simulink model "hydro2pumps_iov1"  (Simulink 7.4)
settings: Solver=ode1  StartTime=0.0  StopTime=inf  FixedStep=0.5  RelTol=1e-3  AbsTol=1e-6
libraries: hydro2pumps_lib x1
settings Model: Creator=dmedonza  LastModifiedBy=student
settings DataIOCC: LimitDataPoints=off  SignalLoggingName=sigsOut
settings OptimizationCC: BooleanDataType=off
settings DebuggingCC: SaveWithParameterizedLinksMsg=none  SignalResolutionControl=TryResolveAllWithWarning  SolverPrmCheckMsg=none  MultiTaskDSMMsg=warning  MultiTaskCondExecSysMsg=none  StrictBusMsg=None
settings HardwareCC: TargetUnknown=on
settings RTWCC: TemplateMakefile=grt_vc.tmf  IncludeERTFirstTime=on

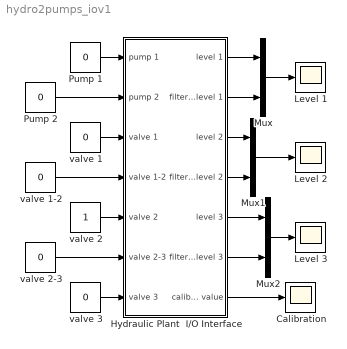
== system hydro2pumps_iov1 ==
  Calibration : Scope
      settings: TickLabels=on  TimeRange=20  YMin=0  YMax=100  SaveName=l3  DataFormat=Array
  Hydraulic Plant  I/O Interface : Subsystem
      mask Display: disp('Two Pumps\nHydraulic\nPlant\nI/O Interface')
  Level 1 : Scope
      settings: TickLabels=on  TimeRange=20  YMin=0  YMax=100  SaveName=l1  DataFormat=Array
  Level 2 : Scope
      settings: TickLabels=on  TimeRange=20  YMin=0  YMax=100  SaveName=l2  DataFormat=Array
  Level 3 : Scope
      settings: TickLabels=on  TimeRange=20  YMin=0  YMax=100  SaveName=lx  DataFormat=Array
  Mux : Mux  Inputs=2
  Mux1 : Mux  Inputs=2
  Mux2 : Mux  Inputs=2
  Pump 1 : Constant  Value=0  OutDataType=sfix(16)  OutScaling=2^0
  Pump 2 : Constant  Value=0  OutDataType=sfix(16)  OutScaling=2^0
  "valve 1 " : Constant  Value=0  OutDataType=sfix(16)  OutScaling=2^0
  valve 1-2 : Constant  Value=0  OutDataType=sfix(16)  OutScaling=2^0
  valve 2 : Constant  OutDataType=sfix(16)  OutScaling=2^0
  valve 2-3 : Constant  Value=0  OutDataType=sfix(16)  OutScaling=2^0
  valve 3 : Constant  Value=0  OutDataType=sfix(16)  OutScaling=2^0
  wires:
  Mux/1 -> Level 1/1
  Mux2/1 -> Level 3/1
  Pump 1/1 -> Hydraulic Plant  I/O Interface/1(pump 1)
  Pump 2/1 -> Hydraulic Plant  I/O Interface/2(pump 2)
  "valve 1 "/1 -> Hydraulic Plant  I/O Interface/3(valve 1)
  valve 1-2/1 -> Hydraulic Plant  I/O Interface/4(valve 1-2)
  valve 2/1 -> Hydraulic Plant  I/O Interface/5(valve 2)
  valve 2-3/1 -> Hydraulic Plant  I/O Interface/6(valve 2-3)
  valve 3/1 -> Hydraulic Plant  I/O Interface/7(valve 3)
  Hydraulic Plant  I/O Interface/1(level 1) -> Mux/1
  Hydraulic Plant  I/O Interface/2(filtered level 1) -> Mux/2
  Hydraulic Plant  I/O Interface/3(level 2) -> Mux1/1
  Hydraulic Plant  I/O Interface/4(filtered level 2) -> Mux1/2
  Hydraulic Plant  I/O Interface/5(level 3) -> Mux2/1
  Hydraulic Plant  I/O Interface/6(filtered level 3) -> Mux2/2
  Hydraulic Plant  I/O Interface/7(calibration value) -> Calibration/1
  Mux1/1 -> Level 2/1

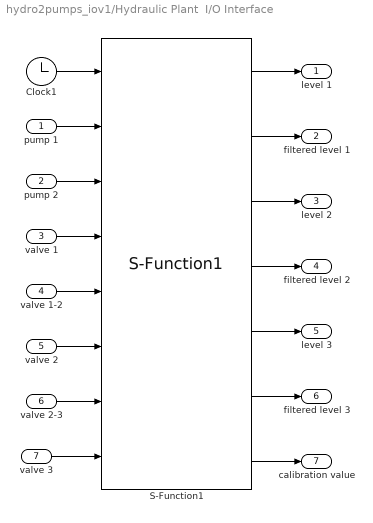
== system hydro2pumps_iov1/Hydraulic Plant  I/O Interface ==
  pump 1 : Inport  OutDataType=sfix(16)  OutScaling=2^0
  pump 2 : Inport  Port=2  OutDataType=sfix(16)  OutScaling=2^0
  valve 1 : Inport  Port=3  OutDataType=sfix(16)  OutScaling=2^0
  valve 1-2 : Inport  Port=4  OutDataType=sfix(16)  OutScaling=2^0
  valve 2 : Inport  Port=5  OutDataType=sfix(16)  OutScaling=2^0
  valve 2-3 : Inport  Port=6  OutDataType=sfix(16)  OutScaling=2^0
  valve 3 : Inport  Port=7  OutDataType=sfix(16)  OutScaling=2^0
  Clock1 : Clock
      settings: Decimation=10
  S-Function1 : hydro2pumps_lib/S-Function1  Priority=1  com_port=COM4  Ts=0.5  events_ot=2  rd_timeout=250  matlab_prior=ABOVE_NORMAL_PRIORITY  warning=on  printout=off
  level 1 : Outport
  filtered level 1 : Outport  Port=2
  level 2 : Outport  Port=3
  filtered level 2 : Outport  Port=4
  level 3 : Outport  Port=5
  filtered level 3 : Outport  Port=6
  calibration value : Outport  Port=7
  wires:
  S-Function1/1 -> level 1/1
  S-Function1/2 -> filtered level 1/1
  Clock1/1 -> S-Function1/1
  pump 1/1 -> S-Function1/2
  pump 2/1 -> S-Function1/3
  S-Function1/3 -> level 2/1
  S-Function1/4 -> filtered level 2/1
  S-Function1/5 -> level 3/1
  S-Function1/6 -> filtered level 3/1
  valve 1/1 -> S-Function1/4
  valve 1-2/1 -> S-Function1/5
  valve 2/1 -> S-Function1/6
  valve 2-3/1 -> S-Function1/7
  S-Function1/7 -> calibration value/1
  valve 3/1 -> S-Function1/8
